simulink model "PnO2017"  (R2017b)
settings: Solver=FixedStepAuto  StartTime=0.0  StopTime=10.0  FixedStep=5e-6  RelTol=1e-3
libraries: powerlib x10, re_lib x1, powerlib_meascontrol x1
settings Model: Creator=ivana  LastModifiedBy=ivana
settings DataIOCC: ReturnWorkspaceOutputs=on
settings DebuggingCC: UnconnectedInputMsg=none  UnconnectedOutputMsg=none  UnconnectedLineMsg=none
settings ModelReferenceCC: EnableRefExpFcnMdlSchedulingChecks=off
settings SFSimCC: SimUseLocalCustomCode=on
settings RTWCC: Description=Generic Real-Time Target  RTWUseLocalCustomCode=on

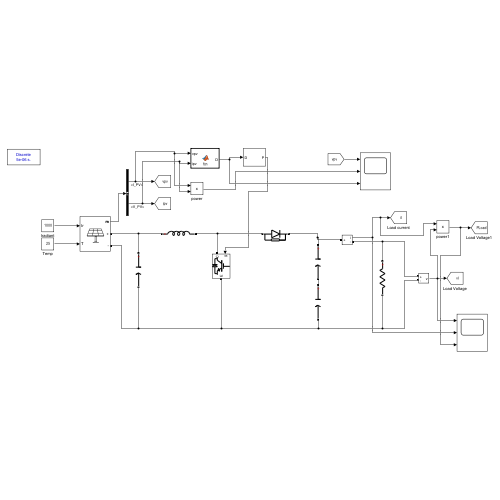
[thumbnail: Simulink's stored preview of the top-level diagram]
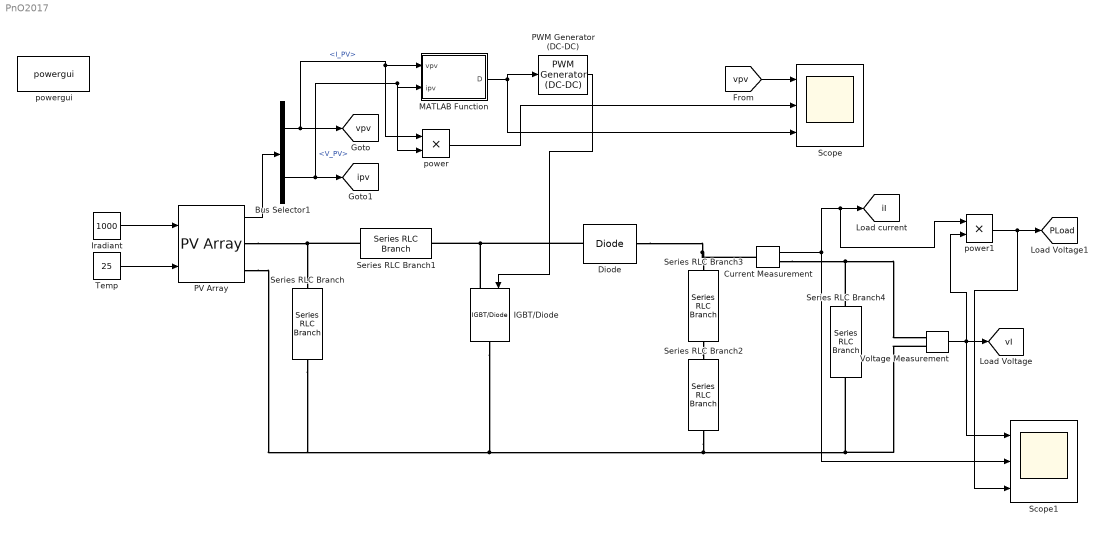
== system PnO2017 ==
  Bus Selector1 : BusSelector  OutputSignals=I_PV,V_PV
  Current Measurement : powerlib/Measurements/Current Measurement  PhasorSimulation=off  OutputType=Complex  PSBequivalent=0
  Diode : powerlib/Power Electronics/Diode  Ron=0.001  Lon=0  Vf=0.8  IC=0  UseSnubber=0  Rs=500  Cs=250e-9  Measurements=off
  IGBT/Diode : powerlib/Power Electronics/IGBT//Diode  Ron=1e-3  Rs=1e5  Cs=inf  Measurements=off
  Iradiant : Constant  Value=1000  VectorParams1D=off
  MATLAB Function : MATLAB Function  TreatAsAtomicUnit=on
  PV Array : re_lib/Solar/PV Array  Npar=64  Nser=5  PlotType=array @ 1000 W/m2 & specified temperatures  S_vec="[ 1000  500  100 ]"  Temp_C_vec="[ 45 25  ]"  ModuleName=SunPower SPR-315E-WHT-D  PlotWhenSelected=off  Pm=315.072  Ncell=96  Voc=64.6  Isc=6.14  Vm=54.7  Im=5.76  beta_Voc_pc=-0.2727  alpha_Isc_pc=0.061743  beta_Voc=-0.17616  alpha_Isc=0.003791  IL=6.1461  I0=6.5067e-12  nI=0.95071  Rsh=430.0666  Rs=0.43041  RobustModel=off  RobustCellTemperature=313.3991  BAL=on  Tc=1e-6  Tfilter=5e-5
  PWM Generator (DC-DC) : powerlib_meascontrol/Pulse & Signal Generators/PWM Generator (DC-DC)  Fsw=5000  Ts=5e-6
  Scope : Scope  NumInputPorts=3
  Scope1 : Scope  NumInputPorts=3
  Series RLC Branch : powerlib/Elements/Series RLC Branch  LConnTagsString=__new0  RConnTagsString=__new0  BranchType=C  Resistance=1  Inductance=1e-3  SetiL0=off  InitialCurrent=0  Capacitance=100e-6  Setx0=off  InitialVoltage=0  Measurements=None
  Series RLC Branch1 : powerlib/Elements/Series RLC Branch  LConnTagsString=__new0  RConnTagsString=__new0  BranchType=L  Resistance=1  Inductance=5e-3  SetiL0=off  InitialCurrent=0  Capacitance=100e-6  Setx0=off  InitialVoltage=0  Measurements=None
  Series RLC Branch2 : powerlib/Elements/Series RLC Branch  LConnTagsString=__new0  RConnTagsString=__new0  BranchType=C  Resistance=1  Inductance=5e-3  SetiL0=off  InitialCurrent=0  Capacitance=12000e-6  Setx0=off  InitialVoltage=0  Measurements=None
  Series RLC Branch3 : powerlib/Elements/Series RLC Branch  LConnTagsString=__new0  RConnTagsString=__new0  BranchType=C  Resistance=1  Inductance=5e-3  SetiL0=off  InitialCurrent=0  Capacitance=12000e-6  Setx0=off  InitialVoltage=0  Measurements=None
  Series RLC Branch4 : powerlib/Elements/Series RLC Branch  LConnTagsString=__new0  RConnTagsString=__new0  BranchType=R  Resistance=20  Inductance=5e-3  SetiL0=off  InitialCurrent=0  Capacitance=12000e-6  Setx0=off  InitialVoltage=0  Measurements=None
  Temp : Constant  Value=25
  Voltage Measurement : powerlib/Measurements/Voltage Measurement  PhasorSimulation=off  OutputType=Complex  PSBequivalent=0
  power : Product
  power1 : Product
  powergui : powerlib/powergui  Priority=1  SimulationMode=Discrete  SampleTime=5e-6  frequency=60  Iterations=50  frequencyindice=0  Pbase=100e6  ErrMax=1e-4  UnitsV=kV  UnitsW=MW  buscounter=0  FunctionMessages=off  echomessages=off  EnableUseOfTLC=off  CurrentSourceSwitches=off  DisableSnubberDevices=off  DisableRonSwitches=off  DisableVfSwitches=off  DisplayEquations=off  AutomaticDiscreteSolvers=off  SolverType=Tustin/Backward Euler (TBE)  Interpol=off  ExternalGateDelay=off  methode=off  Ts=100  x0status=blocks  SPID=on  SwTol=0  HookPort=off  NonlinearTolerance=1e-4  nMaxIteration=100  ContinueOnMaxIteration=off  RestoreLinks=warning  ResistiveCurrentMeasurement=off  Frange=[0:2:500]  Ylog=off  Xlog=on  ShowGrid=off  save=off  variable=ZData  structure=0  ZoomFFT=off  StartTime=0.0  cycles=1  DisplayStyle=1  fundamental=60  FreqAxis=off  MaxFrequency=1000  frequencyindicesteady=1  RmsSteady=1  display=off
  tag scope: PLoad=global, iI=global, ipv=global, vI=global, vpv=global
  wires:
  Iradiant/1 -> PV Array/1
  Temp/1 -> PV Array/2
  PV Array/1 -> Bus Selector1/1
  Bus Selector1/1 -> power/1, MATLAB Function/1(vpv), [vpv]  "<I_PV>"
  Bus Selector1/2 -> power/2, MATLAB Function/2(ipv), [ipv]  "<V_PV>"
  Voltage Measurement/1 -> Scope1/1, power1/2, [vI]
  Current Measurement/1 -> power1/1, [iI], Scope1/2
  PWM Generator (DC-DC)/1 -> IGBT/Diode/1
  [vpv] -> Scope/1
  power/1 -> Scope/2
  MATLAB Function/1(D) -> PWM Generator (DC-DC)/1, Scope/3
  power1/1 -> Scope1/3, [PLoad]
  connections:
  PV Array/RConn1 -- Series RLC Branch/LConn1 -- Series RLC Branch1/LConn1
  IGBT/Diode/LConn1 -- Diode/LConn1 -- Series RLC Branch1/RConn1
  Series RLC Branch4/LConn1 -- Voltage Measurement/LConn1 -- Current Measurement/RConn1
  Series RLC Branch3/RConn1 -- Series RLC Branch2/LConn1
  Series RLC Branch2/RConn1 -- PV Array/RConn2 -- Series RLC Branch/RConn1 -- IGBT/Diode/RConn1 -- Voltage Measurement/LConn2 -- Series RLC Branch4/RConn1
  Diode/RConn1 -- Current Measurement/LConn1 -- Series RLC Branch3/LConn1

== matlab function PnO2017/MATLAB Function ==
  data: vpv input; D output; ipv input
function D = fcn(vpv, ipv)
    % Initialize constants and persistent variables
    persistent Vold Pold Dold
    Dinit = 0.4;
    Dmax = 0.9;
    Dmin = 0.1;
    deltaD = 20e-6;
    
    % Initialize persistent variables on first call
    if isempty(Vold)
        Vold = 0;
        Pold = 0;
        Dold = Dinit;
    end
    
    % Calculate current power and changes in voltage and power
    P = vpv * ipv;
    dV = vpv - Vold;
    dP = P - Pold;
    
    % P&O Algorithm Implementation
    if dP ~= 0
        if dP < 0
            D = Dold - deltaD * sign(dV);
        else
            D = Dold + deltaD * sign(dV);
        end
    else
        D = Dold;
    end
    
    % Ensure D stays within set limits
    if D > Dmax
        D = Dmax;
    elseif D < Dmin
        D = Dmin;
    end
    
    % Update persistent variables
    Dold = D;
    Vold = vpv;
    Pold = P;
end
